simulink model "Model_LAB3_Complete"  (R2024b)
settings: Solver=ode45  StartTime=0.0  StopTime=5  RelTol=1e-2
values from neighbouring files (symbols this model uses):
  pulse2deg = 360/2000    (= 0.18)    [Plant_ModelParameters.m]
undefined symbols (not defined in the file or in its folder): sens
settings Model: Creator=Federico Bergami  LastModifiedBy=Buton

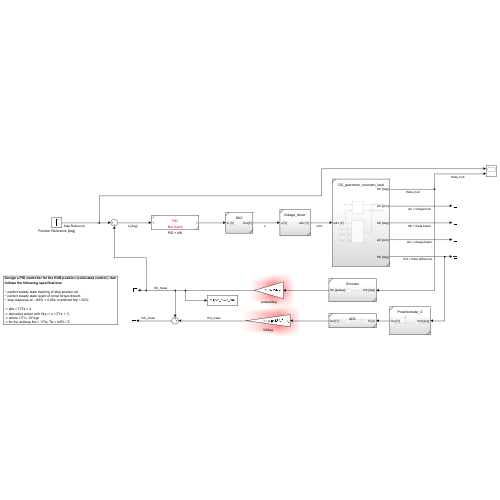
[thumbnail: Simulink's stored preview of the top-level diagram]
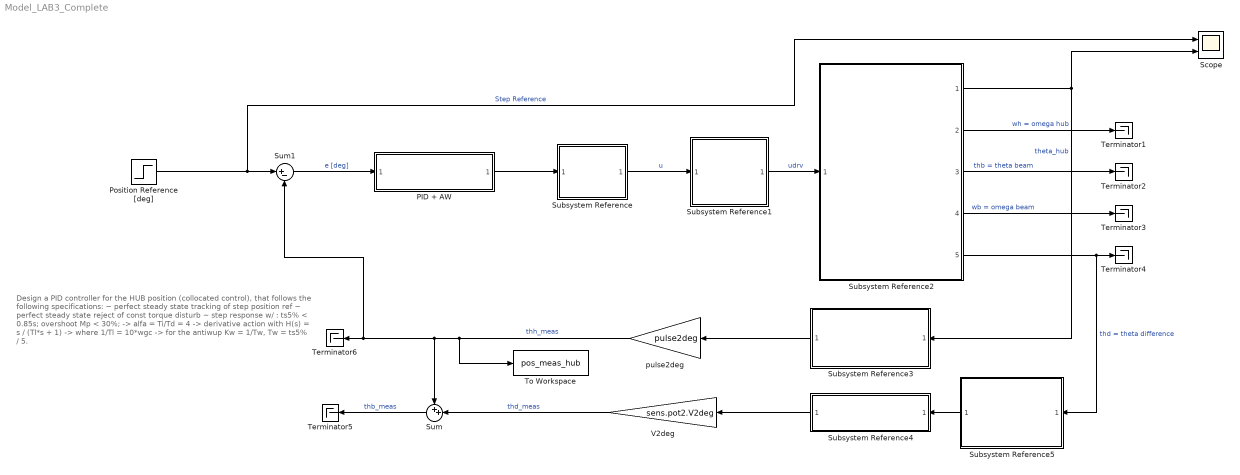
== system Model_LAB3_Complete ==
  note: Design a PID controller for the HUB position (collocated control), that
      | follows the following specifications:
      |
      | ~ perfect steady state tracking of step position ref
      | ~ perfect steady state reject of const torque disturb
      | ~ step response w/ : ts5% < 0.85s; overshoot Mp < 30%;
      |
      | -> alfa = Ti/Td = 4
      | -> derivative action with H(s) = s / (Tl*s + 1)
      | -> where 1/Tl = 10*wgc
      | -> for the antiwup Kw = 1/Tw, Tw = ts5% / 5.
  PID + AW : Subsystem  ReferencedSubsystem=PID
  Position Reference [deg] : Step  Time=0  After=50  SampleTime=0
  Scope : Scope  NumInputPorts=2
  Subsystem Reference : Subsystem  ReferencedSubsystem=DAC
  Subsystem Reference1 : Subsystem  ReferencedSubsystem=Voltage_driver
  Subsystem Reference2 : Subsystem  ReferencedSubsystem=DC_gearmotor_resonant_load
  Subsystem Reference3 : Subsystem  ReferencedSubsystem=Encoder
  Subsystem Reference4 : Subsystem  ReferencedSubsystem=ADC
  Subsystem Reference5 : Subsystem  ReferencedSubsystem=Potentiometer_2
  Sum : Sum  Inputs=++|
  Sum1 : Sum  Inputs=|+-
  Terminator{1..6} (6 alike) : Terminator
  To Workspace : ToWorkspace  VariableName=pos_meas_hub  SaveFormat=Timeseries  SampleTime=-1
  V2deg : Gain  Gain=sens.pot2.V2deg
  pulse2deg : Gain  Gain=pulse2deg
  wires:
  Sum/1 -> Terminator5/1  "thb_meas"
  Subsystem Reference/1 -> Subsystem Reference1/1  "u"
  pulse2deg/1 -> To Workspace/1, Sum/1, Sum1/2, Terminator6/1  "thh_meas"
  Subsystem Reference3/1 -> pulse2deg/1
  Subsystem Reference2/5 -> Subsystem Reference5/1, Terminator4/1  "thd = theta difference"
  V2deg/1 -> Sum/2  "thd_meas"
  Subsystem Reference1/1 -> Subsystem Reference2/1  "udrv"
  Subsystem Reference2/4 -> Terminator3/1  "wb = omega beam"
  Subsystem Reference2/1 -> Scope/2, Subsystem Reference3/1  "theta_hub"
  Subsystem Reference2/2 -> Terminator1/1  "wh = omega hub"
  Subsystem Reference5/1 -> Subsystem Reference4/1
  PID + AW/1 -> Subsystem Reference/1
  Subsystem Reference2/3 -> Terminator2/1  "thb = theta beam"
  Subsystem Reference4/1 -> V2deg/1
  Sum1/1 -> PID + AW/1  "e [deg]"
  Position Reference [deg]/1 -> Scope/1, Sum1/1  "Step Reference"
